simulink model "DirectedEventBroadCast"  (R2020b)
settings: Solver=VariableStepAuto  StartTime=0.0  StopTime=10.0  RelTol=1e-3
settings Model: Creator=apple  LastModifiedBy=apple

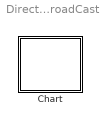
== system DirectedEventBroadCast ==
  Chart : Stateflow chart  TreatAsAtomicUnit=on

== stateflow chart DirectedEventBroadCast/Chart ==
  state A [parallel]
    en:fprintf("Entry A");x = 1;
    settings: executionOrder=1
    state A1
      en:fprintf("Entry A1");
      du:fprintf("During A1");
      ex:fprintf("Exit A1");
    state A2
      en:fprintf("Entry A2");
      du:fprintf("During A2");
      ex:fprintf("Exit A2");
    (default) -> A1
    A1 -> A2 : [x == 1]{send(E_one,B);}
    A2 -> A1 : E_two
  state B [parallel]
    en:fprintf("Entry B");
    settings: executionOrder=2
    state B1
      en:fprintf("Entry B1");
      du:fprintf("During B1");
      ex:fprintf("Exit B1");
    state B2
      en:fprintf("Entry B2");
      du:fprintf("During B2");
      ex:fprintf("Exit B2");
    (default) -> B1
    B1 -> B2 : E_one
    B2 -> B1 : E_two
  data: x local
  events: E_two local FUNCTION_CALL_EVENT; E_one local FUNCTION_CALL_EVENT
